simulink model "model_target"  (R2021a)
settings: Solver=FixedStepDiscrete  StartTime=0.0  StopTime=inf  FixedStep=100  RelTol=1e-3
PreLoadFcn:
  | ip_addr = [202,120,40,8]; role_type = 0; role_tag = 01; role_id = 0002;
  | disp("NOUSE This is drone_static model instance 0001\n");
PreSaveFcn:
  | ip_addr = [202,120,40,8]; role_type = 0; role_tag = 01; role_id = 0002;
settings Model: Creator=FJJ  LastModifiedBy=FJJ
settings SFSimCC: SimUserSources=drone_util.c
settings RTWCC: CustomSource=drone_util.c

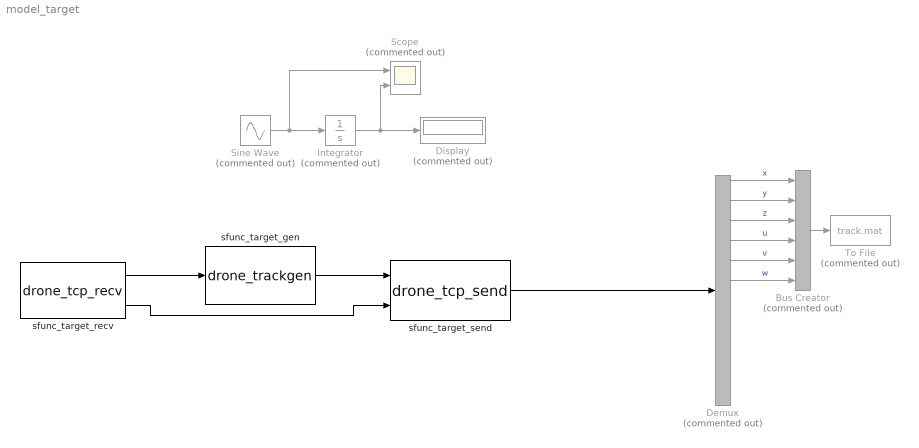
== system model_target ==
  Bus Creator : BusCreator  Commented=on  Inputs=6
  Demux : Demux  Commented=on  Outputs=12
  Display : Display  Commented=on
  Integrator : Integrator  Commented=on
  Scope : Scope  Commented=on  NumInputPorts=2
  Sine Wave : Sin  Commented=on  SampleTime=0
  To File : ToFile  Commented=on  Filename=track.mat  SaveFormat=Timeseries
  sfunc_target_gen : S-Function  FunctionName=drone_trackgen  Parameters=int32(role_type),int32(role_tag),int32(role_id)  SFunctionModules=drone_trackgen_wrapper drone_util  SFunctionDeploymentMode=off  EnableBusSupport=off  mask(S-Function Builder){}
      mask help: Simulink:masks:SFunctionBuilder_MD
      mask init:
      | val = [[.9  0.75 0.75 1 1 .9 .9 1]',[1 1 0.75 0.75 .9 .9 1 .9]'];try , sys = get_param(gcb,'SfunBuilderFcnName');if isempty(sys), sys = get_param(gcb,'FunctionName'); end,catch, sys = get_param(gcb,'FunctionName'); end
      settings: CopyFcn=set_param(gcbh,'LinkStatus','none')  OpenFcn=sfunctionwizard(gcbh)
      mask Display:
      | plot(val(:,1),val(:,2))
      | disp(sys)
      | port_label('input',1,'in')
      | port_label('output',1,'out')
  sfunc_target_recv : S-Function  FunctionName=drone_tcp_recv  Parameters=uint8(ip_addr),int32(30608),int32(role_type),int32(role_tag),int32(role_id)  SFunctionModules=drone_tcp_recv_wrapper drone_util  SFunctionDeploymentMode=off  EnableBusSupport=off  mask(S-Function Builder){}
      mask help: Simulink:masks:SFunctionBuilder_MD
      mask init: same as model_target/sfunc_target_gen
      settings: CopyFcn=set_param(gcbh,'LinkStatus','none')  OpenFcn=sfunctionwizard(gcbh)
      mask Display:
      | plot(val(:,1),val(:,2))
      | disp(sys)
      | port_label('output',1,'out')
      | port_label('output',2,'received')
  sfunc_target_send : S-Function  FunctionName=drone_tcp_send  Parameters=uint8(ip_addr),int32(30608),int32(role_type),int32(role_tag),int32(role_id)  SFunctionModules=drone_tcp_send_wrapper drone_util  SFunctionDeploymentMode=off  EnableBusSupport=off  mask(S-Function Builder){}
      mask help: Simulink:masks:SFunctionBuilder_MD
      mask init: same as model_target/sfunc_target_gen
      settings: CopyFcn=set_param(gcbh,'LinkStatus','none')  OpenFcn=sfunctionwizard(gcbh)
      mask Display:
      | plot(val(:,1),val(:,2))
      | disp(sys)
      | port_label('input',1,'u0')
      | port_label('input',2,'received')
      | port_label('output',1,'y0')
  wires:
  sfunc_target_send/1 -> Demux/1
  Demux/1 -> Bus Creator/1  "x"
  Demux/2 -> Bus Creator/2  "y"
  Demux/3 -> Bus Creator/3  "z"
  Demux/4 -> Bus Creator/4  "u"
  Demux/5 -> Bus Creator/5  "v"
  Demux/6 -> Bus Creator/6  "w"
  Bus Creator/1 -> To File/1
  Sine Wave/1 -> Integrator/1, Scope/1
  Integrator/1 -> Scope/2, Display/1
  sfunc_target_recv/2 -> sfunc_target_send/2
  sfunc_target_recv/1 -> sfunc_target_gen/1
  sfunc_target_gen/1 -> sfunc_target_send/1
